simulink library "ltvlib_20b"  (R2020b)
settings: Solver=VariableStepAuto  StartTime=0.0  StopTime=10.0  RelTol=1e-3
undefined symbols (not defined in the file or in its folder): A, B, C, D, K, L, x0
libraries: $bdroot x10
settings Model: Creator=jyotbuch  LastModifiedBy=Jyot Buch
settings DataIOCC: ReturnWorkspaceOutputs=off
settings DebuggingCC: ArithmeticOperatorsInVariantConditions=warning
settings SFSimCC: CustomCodeUndefinedFunction=UseInterfaceOnly

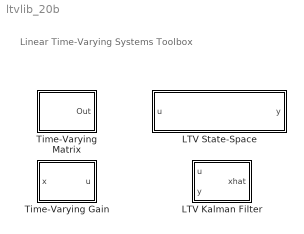
== system ltvlib_20b ==
  note: Linear Time-Varying Systems Toolbox
  LTV Kalman Filter : Subsystem  mask(Linear Time-Varying Kalman Filter){A=A, B=B, C=C, D=D, xhat0=0, L=L}
      mask prompts: A "A(t):"; B "B(t):"; C "C(t):"; D "D(t):"; xhat0 "Estimator Initial Condition:"; L "Kalman Gain:"
      mask help:
      | Outputs the state estimates by using the following equations,
      |
      | dxhat(t)/dt = A(t) xhat(t) + B(t) u(t) + L(t) (y(t) - yhat(t))
      |       yhat(t) = C(t) xhat(t) + D(t) u(t)
      |
      | Where, xhat(t) is an estimated state, u(t) is an input, y(t) is an output, yhat(t) is an estimated output and L(t) is a Kalman Gain which is computed offline. Estimator initial condition xhat0 is required.
      mask init:
      | A = tvmat(A);
      | B = tvmat(B);
      | C = tvmat(C);
      | D = tvmat(D);
      | L = tvmat(L);
      settings: OpenFcn=open_system(gcb,'Mask');
  LTV State-Space : Subsystem  mask(Time-Varying State-Space System){A=A, B=B, C=C, D=D, x0=x0}
      mask prompts: A "A(t):"; B "B(t):"; C "C(t):"; D "D(t):"; x0 "Initial Conditions:"
      mask help:
      | Linear Time-Varying System State-Space Model is given by,
      |
      | dx/dt = A(t) x(t) + B(t) u(t)
      |    y(t) = C(t) x(t) + D(t) u(t)
      |
      | Where, A(t), B(t), C(t), D(t) are time-varying matrices.
      | x(t) is a state, u(t) is an input and y(t) is an output.
      mask init:
      | A = tvmat(A);
      | B = tvmat(B);
      | C = tvmat(C);
      | D = tvmat(D);
      settings: OpenFcn=open_system(gcb,'Mask');
      mask Display:
      | %image(fullfile(resourceroot,'LTV.png'));
      | disp(sprintf('dx(t)/dt = A(t) x(t) + B(t) u(t)\n      y(t) = C(t) x(t) + D(t) u(t)'),'texmode','on');
  Time-Varying Gain : Subsystem  mask(Time-Varying Matrix Gain){K=K}
      mask prompts: K "Gain"
      mask help:
      | Time-Varying matrix gain
      |
      | y(t) = K(t) u(t)
      |
      | Where, u(t) is the input vector with compatible dimensions.
      mask init:
      | K = tvmat(K);
      settings: OpenFcn=open_system(gcb,'Mask');
      mask Display:
      | Gain = get_param(gcb,'K');
      | disp(sprintf('%s(t)',Gain),'texmode','on');
  Time-Varying Matrix : Subsystem  mask(Time-Varying Matrix){M=K, vec1D=on}
      mask prompts: M "Time-Varying Matrix"; vec1D "Interpret vector parameters as 1-D"
      mask help: Output the value of the specified time-varying matrix evaluated at the current simulation time. If the 'Time-Varying Matrix' parameter is M then the output at simulation time t is given by evalt(M,t). If M is a vector and the 'Interpret vector parameters as 1-D' is on, then the output is treated as a 1-D array. Otherwise the output is a matrix with the same dimensions as M.
      mask init:
      | if isequal(M.InterpolationMethod,'Spline') && ...
      |         isempty(M.SplineData)
      |     M = getSplineData(M);
      | end
      | fh = @(t) tvsubs(M,t);
      | szM = size(M);
      | if vec1D==1 && ndims(M)==2 && any(szM==1)
      |     dim = max(szM);
      | else
      |     dim = szM;
      | end
      settings: OpenFcn=open_system(gcb,'Mask');

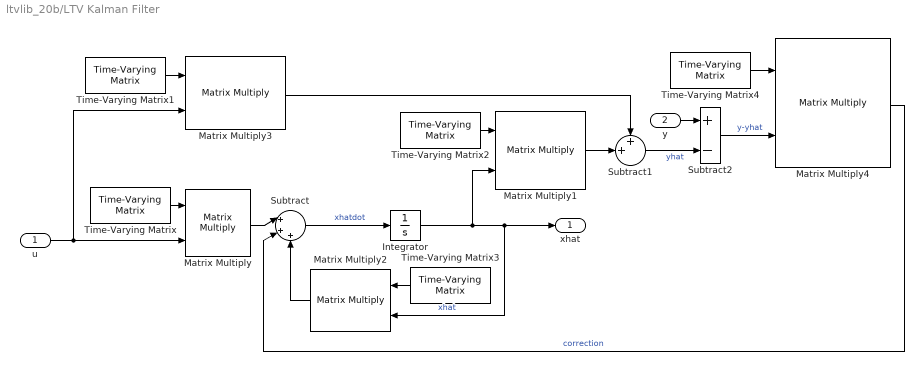
== system ltvlib_20b/LTV Kalman Filter ==
  u : Inport
  y : Inport  Port=2
  Integrator : Integrator  InitialCondition=xhat0
  Matrix Multiply{,1..4} (5 alike) : Product  Multiplication=Matrix(*)
  Subtract : Sum  Inputs=|+++
  Subtract1 : Sum  Inputs=++|
  Subtract2 : Sum  Inputs=+-
  Time-Varying Matrix : $bdroot/Time-Varying Matrix  M=B  vec1D=on
  Time-Varying Matrix1 : $bdroot/Time-Varying Matrix  M=D  vec1D=on
  Time-Varying Matrix2 : $bdroot/Time-Varying Matrix  M=C  vec1D=on
  Time-Varying Matrix3 : $bdroot/Time-Varying Matrix  M=A  vec1D=on
  Time-Varying Matrix4 : $bdroot/Time-Varying Matrix  M=L  vec1D=on
  xhat : Outport  VectorParamsAs1DForOutWhenUnconnected=off
  wires:
  Time-Varying Matrix3/1 -> Matrix Multiply2/1
  Integrator/1 -> Matrix Multiply1/2, xhat/1, Matrix Multiply2/2  "xhat"
  Time-Varying Matrix1/1 -> Matrix Multiply3/1
  Matrix Multiply1/1 -> Subtract1/2
  u/1 -> Matrix Multiply3/2, Matrix Multiply/2
  Matrix Multiply3/1 -> Subtract1/1
  Matrix Multiply2/1 -> Subtract/3
  Time-Varying Matrix2/1 -> Matrix Multiply1/1
  Time-Varying Matrix/1 -> Matrix Multiply/1
  Subtract/1 -> Integrator/1  "xhatdot"
  Subtract1/1 -> Subtract2/2  "yhat"
  Matrix Multiply/1 -> Subtract/1
  y/1 -> Subtract2/1
  Time-Varying Matrix4/1 -> Matrix Multiply4/1
  Subtract2/1 -> Matrix Multiply4/2  "y-yhat"
  Matrix Multiply4/1 -> Subtract/2  "correction"

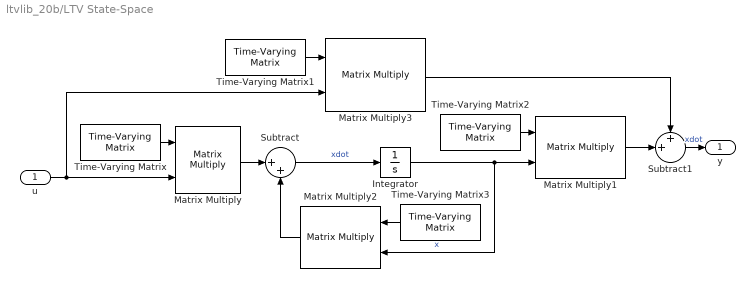
== system ltvlib_20b/LTV State-Space ==
  u : Inport
  Integrator : Integrator  InitialCondition=x0
  Matrix Multiply{,1..3} (4 alike) : Product  Multiplication=Matrix(*)
  Subtract : Sum  Inputs=|++
  Subtract1 : Sum  Inputs=++|
  Time-Varying Matrix : $bdroot/Time-Varying Matrix  M=B  vec1D=on
  Time-Varying Matrix1 : $bdroot/Time-Varying Matrix  M=D  vec1D=on
  Time-Varying Matrix2 : $bdroot/Time-Varying Matrix  M=C  vec1D=on
  Time-Varying Matrix3 : $bdroot/Time-Varying Matrix  M=A  vec1D=on
  y : Outport  VectorParamsAs1DForOutWhenUnconnected=off
  wires:
  Time-Varying Matrix/1 -> Matrix Multiply/1
  u/1 -> Matrix Multiply3/2, Matrix Multiply/2
  Subtract/1 -> Integrator/1  "xdot"
  Matrix Multiply/1 -> Subtract/1
  Integrator/1 -> Matrix Multiply2/2, Matrix Multiply1/2  "x"
  Time-Varying Matrix2/1 -> Matrix Multiply1/1
  Time-Varying Matrix3/1 -> Matrix Multiply2/1
  Matrix Multiply2/1 -> Subtract/2
  Time-Varying Matrix1/1 -> Matrix Multiply3/1
  Matrix Multiply1/1 -> Subtract1/2
  Matrix Multiply3/1 -> Subtract1/1
  Subtract1/1 -> y/1  "xdot"

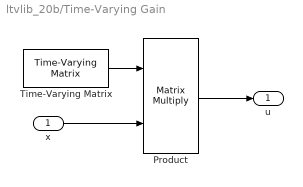
== system ltvlib_20b/Time-Varying Gain ==
  x : Inport
  Product : Product  Multiplication=Matrix(*)
  Time-Varying Matrix : $bdroot/Time-Varying Matrix  M=K  vec1D=off
  u : Outport  VectorParamsAs1DForOutWhenUnconnected=off
  wires:
  x/1 -> Product/2
  Product/1 -> u/1
  Time-Varying Matrix/1 -> Product/1

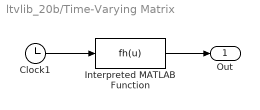
== system ltvlib_20b/Time-Varying Matrix ==
  Clock1 : Clock
  Interpreted MATLAB Function : MATLABFcn  MATLABFcn=fh(u)  OutputDimensions=dim  Output1D=off
  Out : Outport  VectorParamsAs1DForOutWhenUnconnected=off
  wires:
  Interpreted MATLAB Function/1 -> Out/1
  Clock1/1 -> Interpreted MATLAB Function/1
